simulink model "inverter_120_21"  (R2022a)
settings: Solver=VariableStepAuto  StartTime=0.0  StopTime=10.0  RelTol=1e-3
libraries: spsSeriesRLCBranchLib x9, spsIGBTLib x6, simulink x4, spsVoltageMeasurementLib x3, spsDCVoltageSourceLib x1, spsGroundLib x1, spsSawtoothGeneratorLib x1, spsThreePhaseSeriesRLCBranchLib x1, spsThreePhaseVIMeasurementLib x1, spspowerguiLib x1
settings Model: Creator=91894  LastModifiedBy=91894
settings ModelReferenceCC: EnableRefExpFcnMdlSchedulingChecks=off
settings RTWCC: Description=Generic Real-Time Target

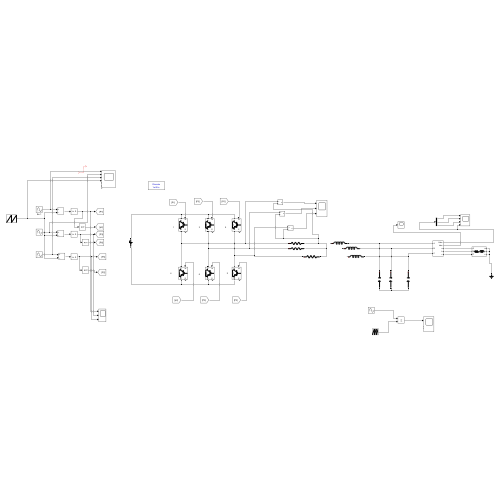
[thumbnail: Simulink's stored preview of the top-level diagram]
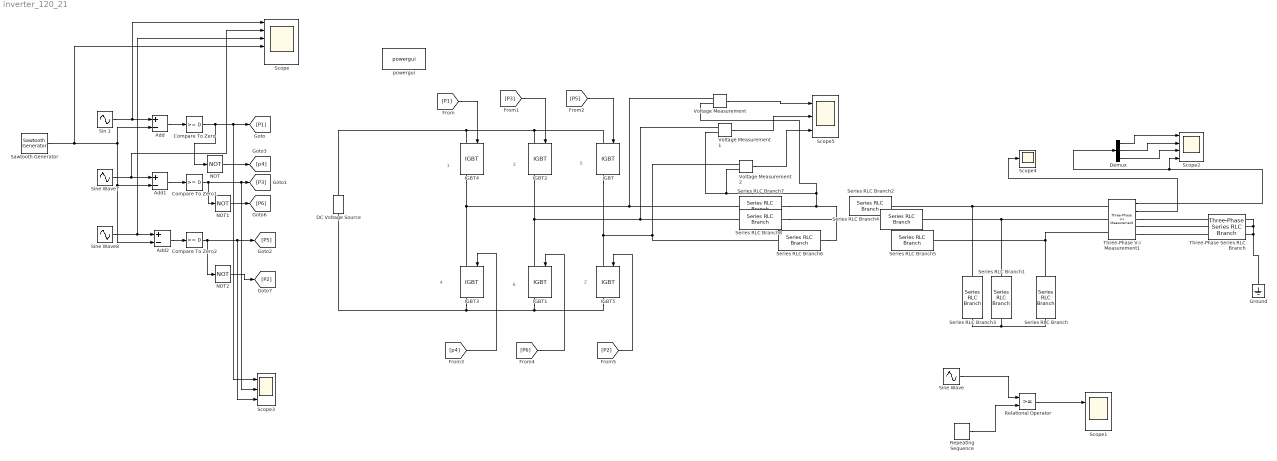
== system inverter_120_21 ==
  note: 2
  note: 6
  note: 4
  note: 5
  note: 3
  note: 1
  Add : Sum  Inputs=+-
  Add1 : Sum  Inputs=+-
  Add2 : Sum  Inputs=+-
  Compare To Zero : simulink/Logic and Bit Operations/Compare To Zero  relop=>=  OutDataTypeStr=boolean
  Compare To Zero1 : simulink/Logic and Bit Operations/Compare To Zero  relop=>=  OutDataTypeStr=boolean  ZeroCross=off
  Compare To Zero2 : simulink/Logic and Bit Operations/Compare To Zero  relop=>=  OutDataTypeStr=boolean
  DC Voltage Source : spsDCVoltageSourceLib/DC Voltage Source  Amplitude=100  Measurements=None
  Demux : Demux  Outputs=3
  Ground : spsGroundLib/Ground  LConnTagsString=a
  IGBT{,1..5} (6 alike) : spsIGBTLib/IGBT  Ron=0.001  Lon=0  Vf=1  Tf=1e-6  Tt=2e-6  IC=0  Rs=1e5  Cs=inf  Measurements=on
  NOT : Logic  Operator=NOT  AllPortsSameDT=off  OutDataTypeStr=boolean
  NOT1 : Logic  Operator=NOT  AllPortsSameDT=off  OutDataTypeStr=boolean
  NOT2 : Logic  Operator=NOT  AllPortsSameDT=off  OutDataTypeStr=boolean
  Relational Operator : RelationalOperator  OutDataTypeStr=boolean  RndMeth=Simplest  InputSameDT=off
  Repeating Sequence : simulink/Sources/Repeating Sequence  rep_seq_t=[0 0.001]  rep_seq_y=[50 100]
  Sawtooth Generator : spsSawtoothGeneratorLib/Sawtooth Generator  Freq=1e4  Phase=0  Ts=0
  Scope : Scope  NumInputPorts=6
  Scope1 : Scope  NumInputPorts=2
  Scope2 : Scope  NumInputPorts=4
  Scope3 : Scope  NumInputPorts=3
  Scope4 : Scope
  Scope5 : Scope  NumInputPorts=3
  Series RLC Branch : spsSeriesRLCBranchLib/Series RLC Branch  LConnTagsString=__new0  RConnTagsString=__new0  BranchType=C  Resistance=1  Inductance=1e-3  SetiL0=off  InitialCurrent=0  Capacitance=6.636e-4  Setx0=off  InitialVoltage=0  Measurements=None
  Series RLC Branch1 : spsSeriesRLCBranchLib/Series RLC Branch  LConnTagsString=__new0  RConnTagsString=__new0  BranchType=C  Resistance=1  Inductance=1e-3  SetiL0=off  InitialCurrent=0  Capacitance=6.636e-4  Setx0=off  InitialVoltage=0  Measurements=None
  Series RLC Branch2 : spsSeriesRLCBranchLib/Series RLC Branch  LConnTagsString=__new0  RConnTagsString=__new0  BranchType=L  Resistance=10  Inductance=3.821e-3  SetiL0=off  InitialCurrent=0  Capacitance=1e-6  Setx0=off  InitialVoltage=0  Measurements=None
  Series RLC Branch3 : spsSeriesRLCBranchLib/Series RLC Branch  LConnTagsString=__new0  RConnTagsString=__new0  BranchType=C  Resistance=1  Inductance=1e-3  SetiL0=off  InitialCurrent=0  Capacitance=6.636e-4  Setx0=off  InitialVoltage=0  Measurements=None
  Series RLC Branch4 : spsSeriesRLCBranchLib/Series RLC Branch  LConnTagsString=__new0  RConnTagsString=__new0  BranchType=L  Resistance=10  Inductance=3.821e-3  SetiL0=off  InitialCurrent=0  Capacitance=1e-6  Setx0=off  InitialVoltage=0  Measurements=None
  Series RLC Branch5 : spsSeriesRLCBranchLib/Series RLC Branch  LConnTagsString=__new0  RConnTagsString=__new0  BranchType=L  Resistance=10  Inductance=3.821e-3  SetiL0=off  InitialCurrent=0  Capacitance=1e-6  Setx0=off  InitialVoltage=0  Measurements=None
  Series RLC Branch6 : spsSeriesRLCBranchLib/Series RLC Branch  LConnTagsString=__new0  RConnTagsString=__new0  BranchType=R  Resistance=1  Inductance=1e-3  SetiL0=off  InitialCurrent=0  Capacitance=1e-6  Setx0=off  InitialVoltage=0  Measurements=None
  Series RLC Branch7 : spsSeriesRLCBranchLib/Series RLC Branch  LConnTagsString=__new0  RConnTagsString=__new0  BranchType=R  Resistance=1  Inductance=1e-3  SetiL0=off  InitialCurrent=0  Capacitance=1e-6  Setx0=off  InitialVoltage=0  Measurements=None
  Series RLC Branch8 : spsSeriesRLCBranchLib/Series RLC Branch  LConnTagsString=__new0  RConnTagsString=__new0  BranchType=R  Resistance=1  Inductance=1e-3  SetiL0=off  InitialCurrent=0  Capacitance=1e-6  Setx0=off  InitialVoltage=0  Measurements=None
  Sin 1 : Sin  Frequency=2*pi*50  SampleTime=0
  Sine Wave : Sin  Amplitude=100  Frequency=50  SampleTime=0
  Sine Wave7 : Sin  Frequency=2*pi*50  Phase=2*pi/3  SampleTime=0
  Sine Wave8 : Sin  Frequency=2*pi*50  Phase=4*pi/3  SampleTime=0
  Three-Phase Series RLC Branch : spsThreePhaseSeriesRLCBranchLib/Three-Phase Series RLC Branch  LConnTagsString=A|B|C  RConnTagsString=A|B|C  BranchType=RL  Resistance=10  Inductance=1e-3  Capacitance=1e-6  Measurements=None
  Three-Phase V-I Measurement1 : spsThreePhaseVIMeasurementLib/Three-Phase V-I Measurement  VoltageMeasurement=phase-to-ground  SetLabelV=off  LabelV=Vabc  Vpu=off  VpuLL=off  CurrentMeasurement=yes  SetLabelI=off  LabelI=Iabc  Ipu=off  Pbase=100e6  Vbase=500e3  OutputType=Complex  PhasorSimulation=off  PSBequivalent=0
  Voltage Measurement : spsVoltageMeasurementLib/Voltage Measurement  PhasorSimulation=off  OutputType=Complex  PSBequivalent=0
  Voltage Measurement1 : spsVoltageMeasurementLib/Voltage Measurement  PhasorSimulation=off  OutputType=Complex  PSBequivalent=0
  Voltage Measurement2 : spsVoltageMeasurementLib/Voltage Measurement  PhasorSimulation=off  OutputType=Complex  PSBequivalent=0
  powergui : spspowerguiLib/powergui  Priority=1  SimulationMode=Discrete  SampleTime=1e-6  frequency=60  Iterations=50  frequencyindice=0  Pbase=100e6  ErrMax=1e-4  UnitsV=kV  UnitsW=MW  buscounter=0  FunctionMessages=off  echomessages=off  EnableUseOfTLC=off  CurrentSourceSwitches=off  DisableSnubberDevices=off  DisableRonSwitches=off  DisableVfSwitches=off  DisplayEquations=off  AutomaticDiscreteSolvers=off  SolverType=Tustin/Backward Euler (TBE)  Interpol=off  ExternalGateDelay=off  methode=off  Ts=100  x0status=blocks  SPID=on  SwTol=0  HookPort=off  NonlinearTolerance=1e-4  nMaxIteration=100  ContinueOnMaxIteration=off  RestoreLinks=warning  ResistiveCurrentMeasurement=off  Frange=[0:2:500]  Ylog=off  Xlog=on  ShowGrid=off  save=off  variable=ZData  structure=0  ZoomFFT=off  StartTime=0.0  cycles=1  DisplayStyle=1  fundamental=60  FreqAxis=off  MaxFrequency=1000  frequencyindicesteady=1  RmsSteady=1  display=off
  wires:
  Sine Wave/1 -> Relational Operator/1
  Repeating Sequence/1 -> Relational Operator/2
  Relational Operator/1 -> Scope1/1
  ? -> ?
  Sin 1/1 -> Scope/1, Add/1
  Sine Wave7/1 -> Scope/2, Add1/1
  Sine Wave8/1 -> Scope/3, Add2/1
  Add2/1 -> Compare To Zero2/1
  Add1/1 -> Compare To Zero1/1
  Add/1 -> Compare To Zero/1
  Sawtooth Generator/1 -> Scope/4, Add2/2, Add1/2, Add/2
  Compare To Zero1/1 -> NOT1/1, Scope3/2, [P3]
  [P5] -> IGBT/1
  [P3] -> IGBT2/1
  [P1] -> IGBT4/1
  [P2] -> IGBT5/1
  [P6] -> IGBT1/1
  [p4] -> IGBT3/1
  Compare To Zero2/1 -> NOT2/1, [P5], Scope3/3
  Compare To Zero/1 -> NOT/1, Scope3/1, [P1]
  NOT/1 -> [p4]
  NOT1/1 -> [P6]
  NOT2/1 -> [P2]
  Demux/1 -> Scope2/1
  Demux/2 -> Scope2/2
  Demux/3 -> Scope2/3
  Three-Phase V-I Measurement1/1 -> Demux/1, Scope2/4
  Three-Phase V-I Measurement1/2 -> Scope4/1
  Voltage Measurement/1 -> Scope5/1
  Voltage Measurement1/1 -> Scope5/2
  Voltage Measurement2/1 -> Scope5/3
  connections:
  IGBT4/LConn1 -- IGBT2/LConn1 -- IGBT/LConn1 -- DC Voltage Source/RConn1
  IGBT5/RConn1 -- IGBT1/RConn1 -- IGBT3/RConn1 -- DC Voltage Source/LConn1
  IGBT4/RConn1 -- Voltage Measurement/LConn1 -- Series RLC Branch7/LConn1 -- IGBT3/LConn1
  IGBT2/RConn1 -- Voltage Measurement1/LConn1 -- Series RLC Branch8/LConn1 -- IGBT1/LConn1
  IGBT/RConn1 -- Voltage Measurement2/LConn1 -- Series RLC Branch6/LConn1 -- IGBT5/LConn1
  Series RLC Branch3/LConn1 -- Series RLC Branch2/RConn1 -- Three-Phase V-I Measurement1/LConn1
  Series RLC Branch1/LConn1 -- Three-Phase V-I Measurement1/LConn2 -- Series RLC Branch4/RConn1
  Series RLC Branch/LConn1 -- Three-Phase V-I Measurement1/LConn3 -- Series RLC Branch5/RConn1
  Series RLC Branch3/RConn1 -- Series RLC Branch1/RConn1 -- Series RLC Branch/RConn1
  Three-Phase V-I Measurement1/RConn1 -- Three-Phase Series RLC Branch/LConn1
  Three-Phase V-I Measurement1/RConn2 -- Three-Phase Series RLC Branch/LConn2
  Three-Phase V-I Measurement1/RConn3 -- Three-Phase Series RLC Branch/LConn3
  Three-Phase Series RLC Branch/RConn1 -- Three-Phase Series RLC Branch/RConn2 -- Ground/LConn1 -- Three-Phase Series RLC Branch/RConn3
  Series RLC Branch8/RConn1 -- Series RLC Branch7/RConn1 -- Voltage Measurement1/LConn2 -- Voltage Measurement2/LConn2 -- Voltage Measurement/LConn2 -- Series RLC Branch6/RConn1
